simulink model "example_cgncc16_paper_gtm"  (R2014a)
settings: Solver=ode45  StartTime=0.0  StopTime=10.0  RelTol=1e-3
values from neighbouring files (symbols this model uses):
  G_post = diag([0.592484 180/pi 1 1])    [example_cgncc16_paper.m]    (also in example_gpr_dob_map.m)
  G_pre = diag([1/0.592484 1 1])    [example_cgncc16_paper.m]    (also in example_gpr_dob_map.m)
  NOISE_ENABLE = 0    [example_cgncc16_paper.m]    (also in example_gpr_dob_map.m)
  state_idx = [1 2 3 4]    [example_cgncc16_paper.m]    (also in example_gpr_dob_map.m)
  Ts = 0.02    [example_cgncc16_paper.m]    (also in example_gpr_dob_map.m)
undefined symbols (not defined in the file or in its folder): sys
undefined symbols (not defined in the file): kf, sys_xm_e_gp, sys_xm_e_kf_delta
settings Model: Creator=encore  LastModifiedBy=encore

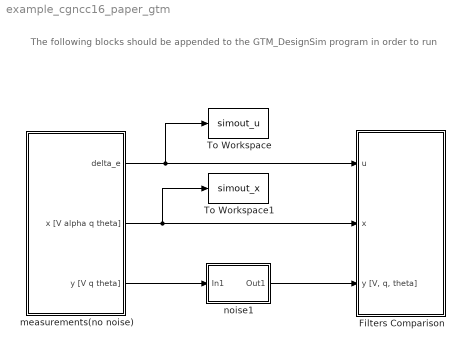
== system example_cgncc16_paper_gtm ==
  note: The following blocks should be appended to the GTM_DesignSim program in order to run
  Filters Comparison : Subsystem
  To Workspace : ToWorkspace  VariableName=simout_u  SaveFormat=Structure With Time  SampleTime=-1
  To Workspace1 : ToWorkspace  VariableName=simout_x  SaveFormat=Structure With Time  SampleTime=-1
  measurements(no noise) : Subsystem
  noise1 : Subsystem
  wires:
  measurements(no noise)/2(x [V alpha q theta]) -> To Workspace1/1, Filters Comparison/2(x)
  measurements(no noise)/1(delta_e) -> To Workspace/1, Filters Comparison/1("u ")
  noise1/1(Out1) -> Filters Comparison/3("y [V, q, theta]")
  measurements(no noise)/3(y [V q theta]) -> noise1/1(In1)

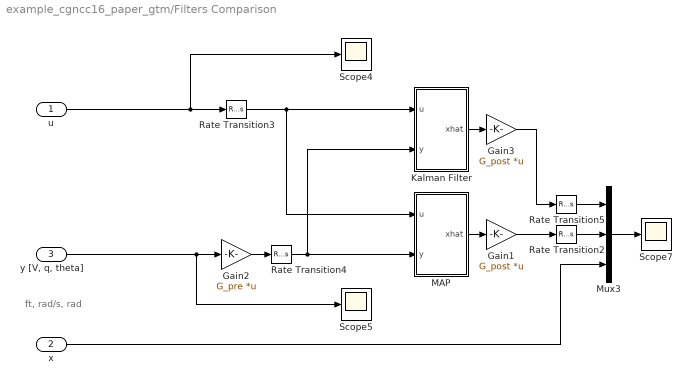
== system example_cgncc16_paper_gtm/Filters Comparison ==
  note: ft, rad/s, rad
  "u " : Inport
  x : Inport  Port=2
  "y [V, q, theta]" : Inport  Port=3
  Gain1 : Gain  Gain=G_post  Multiplication=Matrix(K*u)
  Gain2 : Gain  Gain=G_pre  Multiplication=Matrix(K*u)
  Gain3 : Gain  Gain=G_post  Multiplication=Matrix(K*u)
  Kalman Filter : Subsystem
  MAP : Subsystem  TreatAsAtomicUnit=on  mask{x0=sys_xm_e_gp, Ts=Ts}
      mask prompts: x0 "Initial estimation of the mean of x: x0"; Ts "Sampling period"
  Mux3 : Mux  Inputs=3
  Rate Transition{2..5} (4 alike) : RateTransition
  Scope4 : Scope
      settings: SaveName=scope_u
  Scope5 : Scope
      settings: YMax=80  SaveName=scope_x
  Scope7 : Scope
      settings: TimeRange=4  YMax=80  SaveName=scope_xh
  wires:
  Rate Transition3/1 -> MAP/1(u), Kalman Filter/1(u)
  Mux3/1 -> Scope7/1
  MAP/1(xhat) -> Gain1/1
  Kalman Filter/1(xhat) -> Gain3/1
  "u "/1 -> Scope4/1, Rate Transition3/1
  Rate Transition4/1 -> Kalman Filter/2(y), MAP/2(y)
  Rate Transition5/1 -> Mux3/1
  Rate Transition2/1 -> Mux3/2
  "y [V, q, theta]"/1 -> Gain2/1, Scope5/1
  Gain2/1 -> Rate Transition4/1
  Gain1/1 -> Rate Transition2/1
  Gain3/1 -> Rate Transition5/1
  x/1 -> Mux3/3

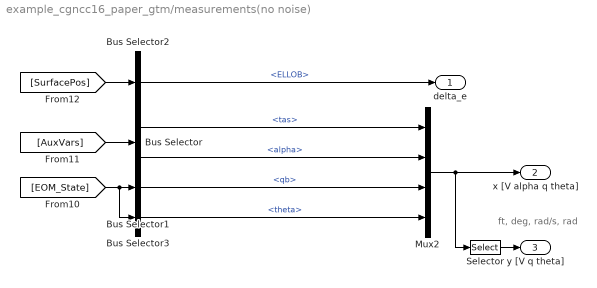
== system example_cgncc16_paper_gtm/measurements(no noise) ==
  note: ft, deg, rad/s, rad
  Bus Selector : BusSelector  OutputSignals=tas,alpha
  Bus Selector1 : BusSelector  OutputSignals=qb
  Bus Selector2 : BusSelector  OutputSignals=ELLOB
  Bus Selector3 : BusSelector  OutputSignals=theta
  Mux2 : Mux
  Selector : Selector  InputPortWidth=numel(state_idx)  Indices=state_idx(state_idx~=rho_idx)
  delta_e : Outport
  x [V alpha q theta] : Outport  Port=2
  y [V q theta] : Outport  Port=3
  wires:
  Bus Selector/2 -> Mux2/2  "<alpha>"
  [EOM_State] -> Bus Selector3/1, Bus Selector1/1
  Bus Selector/1 -> Mux2/1  "<tas>"
  [SurfacePos] -> Bus Selector2/1
  [AuxVars] -> Bus Selector/1
  Bus Selector2/1 -> delta_e/1  "<ELLOB>"
  Bus Selector1/1 -> Mux2/3  "<qb>"
  Mux2/1 -> Selector/1, x [V alpha q theta]/1
  Bus Selector3/1 -> Mux2/4  "<theta>"
  Selector/1 -> y [V q theta]/1

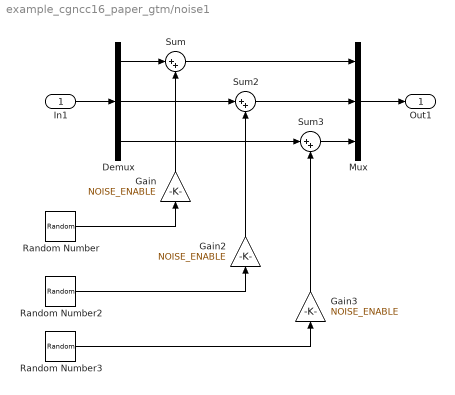
== system example_cgncc16_paper_gtm/noise1 ==
  In1 : Inport
  Demux : Demux  Outputs=3
  Gain : Gain  Gain=NOISE_ENABLE
  Gain2 : Gain  Gain=NOISE_ENABLE
  Gain3 : Gain  Gain=NOISE_ENABLE
  Mux : Mux  Inputs=3
  Random Number : RandomNumber
  Random Number2 : RandomNumber  Variance=0.001
  Random Number3 : RandomNumber  Variance=0.001
  Sum : Sum  Inputs=|++
  Sum2 : Sum  Inputs=|++
  Sum3 : Sum  Inputs=|++
  Out1 : Outport
  wires:
  Random Number3/1 -> Gain3/1
  Random Number/1 -> Gain/1
  Gain3/1 -> Sum3/2
  Gain/1 -> Sum/2
  Random Number2/1 -> Gain2/1
  Demux/1 -> Sum/1
  Demux/3 -> Sum3/1
  Gain2/1 -> Sum2/2
  Mux/1 -> Out1/1
  Sum/1 -> Mux/1
  In1/1 -> Demux/1
  Sum3/1 -> Mux/3
  Sum2/1 -> Mux/2
  Demux/2 -> Sum2/1

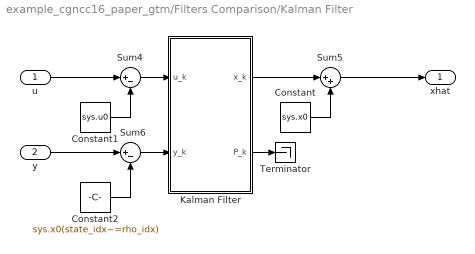
== system example_cgncc16_paper_gtm/Filters Comparison/Kalman Filter ==
  u : Inport
  y : Inport  Port=2
  Constant : Constant  Value=sys.x0
  Constant1 : Constant  Value=sys.u0  SampleTime=Ts
  Constant2 : Constant  Value=sys.x0(state_idx~=rho_idx)  SampleTime=Ts
  Kalman Filter : Subsystem  mask{A=sys.A, B=sys.B, C=sys.C, x0=sys_xm_e_kf_delta, P0=kf.P0, Q=kf.Q, R=kf.R, Ts=Ts}
      mask prompts: A "System matrix A"; B "Input matrix B"; C "Output matrix C"; x0 "Initial estimation of the mean of x: x0"; P0 "Initial estimation of the covariance of x: P0"; Q "Process noise covariance Q"; R "Measurement noise covariance R"; Ts "Sampling period"
  Sum4 : Sum  Inputs=|+-
  Sum5 : Sum  Inputs=|++
  Sum6 : Sum  Inputs=|+-
  Terminator : Terminator
  xhat : Outport
  wires:
  Constant1/1 -> Sum4/2
  u/1 -> Sum4/1
  Sum4/1 -> Kalman Filter/1(u_k)
  Kalman Filter/1(x_k) -> Sum5/1
  Sum6/1 -> Kalman Filter/2(y_k)
  y/1 -> Sum6/1
  Kalman Filter/2(P_k) -> Terminator/1
  Constant/1 -> Sum5/2
  Constant2/1 -> Sum6/2
  Sum5/1 -> xhat/1

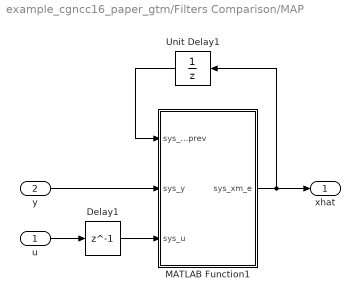
== system example_cgncc16_paper_gtm/Filters Comparison/MAP ==
  u : Inport  OutDataTypeStr=double
  y : Inport  Port=2  OutDataTypeStr=double
  Delay1 : Delay  DelayLength=1  SampleTime=Ts
  MATLAB Function1 : MATLAB Function  TreatAsAtomicUnit=on  SystemSampleTime=Ts
  Unit Delay1 : UnitDelay  InitialCondition=x0  SampleTime=Ts
  xhat : Outport
  wires:
  u/1 -> Delay1/1
  y/1 -> MATLAB Function1/2(sys_y)
  Delay1/1 -> MATLAB Function1/3(sys_u)
  MATLAB Function1/1(sys_xm_e) -> Unit Delay1/1, xhat/1
  Unit Delay1/1 -> MATLAB Function1/1(sys_xm_e_prev)

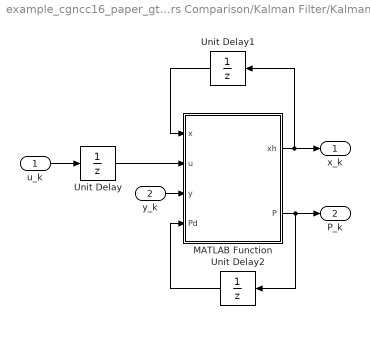
== system example_cgncc16_paper_gtm/Filters Comparison/Kalman Filter/Kalman Filter ==
  u_k : Inport
  y_k : Inport  Port=2
  MATLAB Function : MATLAB Function  TreatAsAtomicUnit=on  SystemSampleTime=Ts
  Unit Delay : UnitDelay  SampleTime=Ts
  Unit Delay1 : UnitDelay  InitialCondition=x0  SampleTime=-1
  Unit Delay2 : UnitDelay  InitialCondition=P0  SampleTime=-1
  x_k : Outport
  P_k : Outport  Port=2
  wires:
  Unit Delay/1 -> MATLAB Function/2(u)
  MATLAB Function/2(P) -> Unit Delay2/1, P_k/1
  u_k/1 -> Unit Delay/1
  Unit Delay1/1 -> MATLAB Function/1(x)
  y_k/1 -> MATLAB Function/3(y)
  MATLAB Function/1(xh) -> Unit Delay1/1, x_k/1
  Unit Delay2/1 -> MATLAB Function/4(Pd)

== matlab function example_cgncc16_paper_gtm/Filters Comparison/Kalman Filter/Kalman Filter/MATLAB Function ==
  data: x input; u input; y input; Pd input; A parameter; B parameter; C parameter; Q parameter; R parameter; xh output; P output
function [xh, P] = kalmanfd(x,u,y,Pd,A,B,C,Q,R)
% x <- x_{k-1}
% u <- u_{k-1}
% y <- y_{k}
%#codegen
fx = A*x+B*u;
hx = C*fx;
F = A;
H = C;
[xh, P] = ekfd(y, fx, hx, F, H, Q, R, Pd);

== matlab function example_cgncc16_paper_gtm/Filters Comparison/MAP/MATLAB Function1 ==
  data: sys_xm_e_prev input; sys_xm_e output double size=size(x0); sys_y input; sys_u input
function sys_xm_e  = GPR_DOB_MAP(sys_xm_e_prev, sys_y,sys_u)
%#codegen
coder.extrinsic('gpr_dob_map');
sys_xm_e = gpr_dob_map(sys_y, sys_u, sys_xm_e_prev);
end
